simulink model "Project2_SimModel"  (R2021b)
settings: Solver=VariableStepAuto  StartTime=0.0  StopTime=10.0  RelTol=1e-3
values from neighbouring files (symbols this model uses):
  As = sys.A    [ObserverDesignWithKalmanFilter.m]
  Bs = sys.B    [ObserverDesignWithKalmanFilter.m]
  Cs = sys.C    [ObserverDesignWithKalmanFilter.m]
  DishObs = ss(A-L*C,[B-L*D, L],eye(2),zeros(2,2),Ts)    [Project2_ObserverDesign.m]    (also in Project2_ObserverDesign_RevisedStateMatrix.m; Project2_ObserverDesign_WithIntegrator.m = ss(A-L*C,[B-L*D, L],eye(3),zeros(3,2),Ts))
  Ds = sys.D    [ObserverDesignWithKalmanFilter.m]
libraries: simulink x1
settings Model: Creator=randy  LastModifiedBy=randy

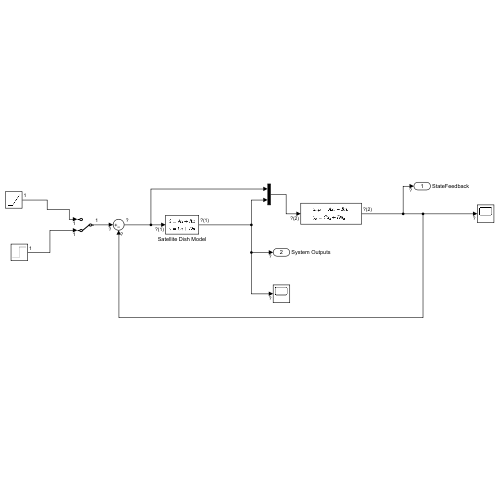
[thumbnail: Simulink's stored preview of the top-level diagram]
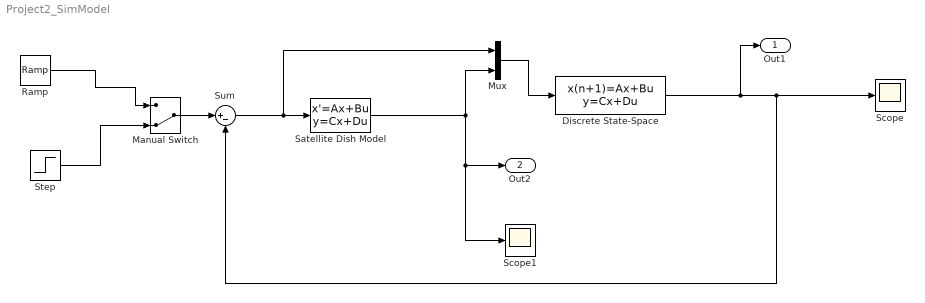
== system Project2_SimModel ==
  Discrete State-Space : DiscreteStateSpace  A=DishObs.A  B=DishObs.B  C=DishObs.C  D=DishObs.D  InitialCondition=2  SampleTime=0.05
  Manual Switch : ManualSwitch  CurrentSetting=0
  Mux : Mux  Inputs=2
  Ramp : simulink/Sources/Ramp  slope=0.78  start=0  InitialOutput=0
  Satellite Dish Model : StateSpace  A=As  B=Bs  C=Cs  D=Ds  InitialCondition=0
  Scope : Scope
  Scope1 : Scope
  Step : Step  After=12.5  SampleTime=0
  Sum : Sum  Inputs=|+-
  Out1 : Outport  SignalName=StateFeedback
  Out2 : Outport  Port=2  SignalName=System Outputs
  wires:
  Sum/1 -> Mux/1, Satellite Dish Model/1
  Discrete State-Space/1 -> Sum/2, Scope/1, Out1/1
  Manual Switch/1 -> Sum/1
  Step/1 -> Manual Switch/2
  Ramp/1 -> Manual Switch/1
  Satellite Dish Model/1 -> Mux/2, Scope1/1, Out2/1
  Mux/1 -> Discrete State-Space/1
